simulink model "CRCL"  (R2020b)
settings: Solver=FixedStepDiscrete  StartTime=0.0  StopTime=inf  FixedStep=0.01  RelTol=1e-3  EnableMultiTasking=on
values from neighbouring files (symbols this model uses):
  calibrationDelayTime_s = 2.0    [CRCL_Dictionary.sldd]
  collisionAngleThreshold_deg = 40.0    [CRCL_Dictionary.sldd]
  collisionVarianceThreshold_g2 = 8.0    [CRCL_Dictionary.sldd]
  cpMaxAbortTime_s = 30.0    [CRCL_Dictionary.sldd]
  cpMaxTipOverAngle_deg = 35.0    [CRCL_Dictionary.sldd]
  cpMinEstDistance_m = 50.0    [CRCL_Dictionary.sldd]
  cpMinEstDistanceGnssBased_m = 200.0    [CRCL_Dictionary.sldd]
  cpMinRiddenTime_s = 15.0    [CRCL_Dictionary.sldd]
  cpMinSpeedRiding_kmh = 10.0    [CRCL_Dictionary.sldd]
  cpNumCrankRevolutionThreshold = 5.0    [CRCL_Dictionary.sldd]
  cpSpeedCond2PositiveSpeedChangeTime_s = 5.0    [CRCL_Dictionary.sldd]
  cpSpeedDerivativeThreshold_kmhs = 0.005    [CRCL_Dictionary.sldd]
  cpTimeOutSpeedCond2_s = 15.0    [CRCL_Dictionary.sldd]
  groundHitEnergyThresholdStanding_g2s2 = 0.02    [CRCL_Dictionary.sldd]
  groundHitTipOverAngleThreshold_deg = 40.0    [CRCL_Dictionary.sldd]
  longAccCompForEulerEstFlag = 0.0    [CRCL_Dictionary.sldd]
  minEnergyStrongHit_g2s2 = 0.1    [CRCL_Dictionary.sldd]
  noMotionAccVarianceThresholdSD_g2 = 0.001    [CRCL_Dictionary.sldd]
  ride1minSpeedSlow_kmh = 4.0    [CRCL_Dictionary.sldd]
  ride2minSpeed_kmh = 8.0    [CRCL_Dictionary.sldd]
  rroMaxSpeed_kmh = 5.0    [CRCL_Dictionary.sldd]
  rroMinGyrX_degs = 20.0    [CRCL_Dictionary.sldd]
  rroMonotonyThreshold_degs = -1.0    [CRCL_Dictionary.sldd]
  rroRollIntegrationAngleThreshold_degs = 20.0    [CRCL_Dictionary.sldd]
  rroUniContinuityThreshold_degs = 15.0    [CRCL_Dictionary.sldd]
  scaleFactorVarianceStrongHit = 2.0    [CRCL_Dictionary.sldd]
  sdoMaxAccVarFreeFall_g2 = 0.06    [CRCL_Dictionary.sldd]
  sdoMaxTipOverAngle_deg = 20.0    [CRCL_Dictionary.sldd]
  sdoMinAccVar_g2 = 8.0    [CRCL_Dictionary.sldd]
  sdoMinGyrXYNorm_degs = 720.0    [CRCL_Dictionary.sldd]
  sdoMinGyrXYNormFreeFall_degs = 100.0    [CRCL_Dictionary.sldd]
  sdoMinOrientationChange_deg = 120.0    [CRCL_Dictionary.sldd]
  sdoScaleFactorOrientationChange = 3.0    [CRCL_Dictionary.sldd]
  stepTime_s = 0.01    [CRCL_Dictionary.sldd]
  strongHitSafetyFactor = 2.5    [CRCL_Dictionary.sldd]
  tipOverAccZFiltTreshold_g = 0.7    [CRCL_Dictionary.sldd]
  tipOverAngleThreshold_deg = 50.0    [CRCL_Dictionary.sldd]
  tipOverMinAccZFiltNoseOver_g = 0.3    [CRCL_Dictionary.sldd]
  tipOverRollPitchRelationNoseOver = 1.5    [CRCL_Dictionary.sldd]
undefined symbols (not defined in the file or in its folder): magnitude
libraries: simulink x17
(part 7 of 8)

== matlab function CRCL/MATLAB Function5 ==
  data: tipOverAngle_deg input; probCollision output; probStrongCollision output; probSoftCollision output; speed_kmh input; accEnergyXY50ms input; accEnergyXY70ms input; accEnergyXY70msLatched input; accVariance70msLatched input; secondCalibDone input; probGroundHit output; accImpulseY input; RollDeriv input; probRd1 output; probRd2 output; probTipOver12 output; probTipOver2 output; speedDerivative input; tipOverAngleTransformedColl output; speedTransformedColl output; speed2sTransformedRd output; speedDerivativeTransformedRd output; accTipOverAngle_deg input; pitch_deg input; roll_deg input; accBfZfilt input; tipOverAngleFusedTransformedTOl output; TipOverAngleAccTransformedTOl output; pitchAngleTransformationTO2 output; pitchRollRelationTransformationTO2 output; accBfZTransformationTO2 output; systemConfig input; cobiHubSetup input; curDuAccZFiltG input
function [probCollision, probStrongCollision, probSoftCollision, ...
    probGroundHit, probRd1, probRd2, probTipOver12, probTipOver2, ...
    tipOverAngleTransformedColl, speedTransformedColl,...
    speed2sTransformedRd, speedDerivativeTransformedRd,...
    tipOverAngleFusedTransformedTOl, TipOverAngleAccTransformedTOl , ...
    pitchAngleTransformationTO2, pitchRollRelationTransformationTO2, ...
    accBfZTransformationTO2] = crashFeatureProbabilityEstimation(tipOverAngle_deg, ...
    speed_kmh, accEnergyXY50ms, accEnergyXY70ms, accEnergyXY70msLatched,...
    accVariance70msLatched, secondCalibDone, ...
    accImpulseY,RollDeriv, speedDerivative, accTipOverAngle_deg, ...
    pitch_deg, roll_deg, accBfZfilt, systemConfig, cobiHubSetup, ...
    curDuAccZFiltG)

persistent i ringBufSpeed2s speed2s_kmh

if isempty(i)
    i = single(1);
    ringBufSpeed2s= single(zeros(20,1));
    speed2s_kmh = single(0);  
end

if mod(i,10) == 0
    ringBufSpeed2s(i/10) = speed_kmh;
    if i == 200
        speed2s_kmh = ringBufSpeed2s(1);
    else
        speed2s_kmh = ringBufSpeed2s(i/10+1);
    end
    if min(ringBufSpeed2s) < speed2s_kmh
        speed2s_kmh = min(ringBufSpeed2s);
    end
end


%% general parameters
strongCollisionSafety = single(3);
softCollisionScale = single(2);


%% probabilistic models
B_groundHit = single([-32.0602312846622;30.8165649192532;0.531118388570848;172.376443479951]);
B_collision = single([-2.87196689910160;-29.6105557448201;-5.00762861256094;241.946430188289]);
B_rd1 = single([-29.0217184513153;8.06889061930136]);
B_rd2 = single([-42.1335668740954;23.9784829246872;9.23975798539886;1.14044463386772]);
%B_tipOver12 = single([-1.371493988037109e+02;68.892066955566400;74.731811523437500]);
B_tipOver12 = single([-32.032394409179690;21.612045288085938;19.315736770629883]);
B_tipOver2 =single([-31.113632202148438;15.738595962524414;10.099098205566406;12.869010925292969]);


%% variable transformation
% CollisionHit and GroundHit
% speed:   'f(x)=1-exp(-speedTransform_c0*x)'
c0_speedTransformColl = 0.125;

speedTransformedColl = 1-expApproxFunc(-c0_speedTransformColl*speed_kmh);

% tipOverAngleSigmoid:
% 'f(x)=1/(1+expApproxFunc(-tipOverTransform_c0*(x-tipOverTransform_c1)))'
tipOverSigmoidTransformColl_c0 = single(0.3);   %0.4
tipOverSigmoidTransformColl_c1 = single(42);    %38

tipOverAngleTransformedColl = 1/(1+expApproxFunc(-tipOverSigmoidTransformColl_c0*(tipOverAngle_deg-tipOverSigmoidTransformColl_c1)));

% TipOverFeature
tipOverSigmoidTransformTol_c0 = single(0.33); %0.5
tipOverSigmoidTransformTol_c1 = single(45); 
noseOverSigmoidTransformTo2_c0 = single(0.1); %0.5
noseOverSigmoidTransformTo2_c1 = single(45); 
noseOverSigmoidAccTransform_c0 = 50;
noseOverSigmoidAccTransform_c1 = 0.3;
noseOverSigmoidPitchRollRelationTransform_c0 = 10;
noseOverSigmoidPitchRollRelationTransform_c1 = 1.5;


tipOverAngleFusedTransformedTOl = 1/(1+expApproxFunc(-tipOverSigmoidTransformTol_c0*(tipOverAngle_deg-tipOverSigmoidTransformTol_c1)));
TipOverAngleAccTransformedTOl = 1/(1+expApproxFunc(-tipOverSigmoidTransformTol_c0*(accTipOverAngle_deg-tipOverSigmoidTransformTol_c1)));
pitchAngleTransformationTO2= 1/(1+expApproxFunc(-noseOverSigmoidTransformTo2_c0*(pitch_deg-noseOverSigmoidTransformTo2_c1)));
pitchRollRelationTransformationTO2 = 1/(1+expApproxFunc(-noseOverSigmoidPitchRollRelationTransform_c0*(abs(pitch_deg)/abs(roll_deg)-noseOverSigmoidPitchRollRelationTransform_c1)));
accBfZTransformationTO2 = 1/(1+expApproxFunc(-noseOverSigmoidAccTransform_c0*(accBfZfilt-noseOverSigmoidAccTransform_c1)));

% RideFeature
%speed(t-2s)
c0_SpeedTransformRd = single(5); 
c1_SpeedTransformRd = single(8);

speed2sTransformedRd = 1./(1+expApproxFunc(-c0_SpeedTransformRd.*(speed2s_kmh-c1_SpeedTransformRd)));

%speed derivative
c0_SpeedDerivativeTransformRd = single(10); 
c1_SpeedDerivativeTransformRd = single(-2.5); 

speedDerivativeTransformedRd = 1./(1+expApproxFunc(-c0_SpeedDerivativeTransformRd.*(speedDerivative-c1_SpeedDerivativeTransformRd)));

%% estimation of crash feature probabilities

if secondCalibDone == 1
    %collision
    if accEnergyXY70ms >= 0.003 && tipOverAngle_deg <= 45
        probCollision = 1 ./ (1 + expApproxFunc(-(B_collision(1) + ...
            tipOverAngleTransformedColl .* B_collision(2) + speedTransformedColl .* ...
            B_collision(3) + accEnergyXY70ms .* B_collision(4)))); %sigmoid function
    else
        probCollision = single(0);
    end

    %strongCollision
    if accEnergyXY70msLatched >= 0.003 && tipOverAngle_deg <= 45 && ...
            accVariance70msLatched >= 12                                    %min variance for strongHits!
        probStrongCollision = 1 ./ (1 + expApproxFunc(-(B_collision(1) + ...
            tipOverAngleTransformedColl .* B_collision(2) + speedTransformedColl .* ...
            B_collision(3) + 1/strongCollisionSafety * accEnergyXY70msLatched .* B_collision(4)))); %sigmoid function
    else
        probStrongCollision = single(0);
    end

    %softCollision
    if accEnergyXY70ms >= 0.003 && tipOverAngle_deg <= 45 && speed_kmh <= 4.5 && ...
            (accImpulseY*RollDeriv >= 0 || accEnergyXY70ms >= 0.015 || tipOverAngle_deg <= 10)  % dismiss fallOver on pedal
        probSoftCollision = 1 ./ (1 + expApproxFunc(-(B_collision(1) + ...
            tipOverAngleTransformedColl .* B_collision(2) + speedTransformedColl .* ...
            B_collision(3) + softCollisionScale * accEnergyXY70ms .* B_collision(4)))); %sigmoid function
    else
        probSoftCollision = single(0);
    end

    %groundHit
    if accEnergyXY50ms >= 0.002 && tipOverAngle_deg >= 35
        probGroundHit = 1 ./ (1 + expApproxFunc(-(B_groundHit(1) + ...
            tipOverAngleTransformedColl .* B_groundHit(2) + speedTransformedColl .* ...
            B_groundHit(3) + accEnergyXY50ms .* B_groundHit(4)))); %sigmoid function
    else
        probGroundHit = single(0);
    end
    
    %tipOver Feature
    if systemConfig == 2 && cobiHubSetup == 2 && curDuAccZFiltG <= 0.75
        probTipOver12 = single(1 ./ (1 + expApproxFunc(-(B_tipOver12(1) + ...
            tipOverAngleFusedTransformedTOl .* B_tipOver12(2) + ...
            TipOverAngleAccTransformedTOl .* B_tipOver12(3)))));
    elseif systemConfig ~= 2 || cobiHubSetup ~= 2
        probTipOver12 = single(1 ./ (1 + expApproxFunc(-(B_tipOver12(1) + ...
            tipOverAngleFusedTransformedTOl .* B_tipOver12(2) + ...
            TipOverAngleAccTransformedTOl .* B_tipOver12(3)))));
    else
        probTipOver12 = single(0);
    end
    if abs(roll_deg) <= 30
        probTipOver2 = single(1 ./ (1 + expApproxFunc(-(B_tipOver2(1) + ...
            pitchAngleTransformationTO2 .* B_tipOver2(2) + ...
            pitchRollRelationTransformationTO2 .* B_tipOver2(3)+ ...
             accBfZTransformationTO2 .* B_tipOver2(4)))));
    else
        probTipOver2 = single(0);
    end
    
else    
    %no Calibration yet
    probCollision = single(0);
    probStrongCollision = single(0);
    probSoftCollision = single(0);
    probGroundHit = single(0);
    probTipOver12 = single(0);
    probTipOver2 = single(0);
end

%Ride Feature
probRd1 = 1./(1+expApproxFunc(-(B_rd1(1)+B_rd1(2).*speed_kmh)));
probRd2 = 1 ./ (1 + expApproxFunc(-(B_rd2(1) + speed2sTransformedRd .* B_rd2(2) + ...
    speedDerivativeTransformedRd .* B_rd2(3) + speed_kmh .* B_rd2(4)))); %sigmoid function


speed2sDebug_kmh = speed2s_kmh;

i = i + 1;
if i >= 201
    i=single(1);
end

end

%approximation for exponential function
function y = expApproxFunc(x_arg)

    denominatorPower = single(1024);
    log2Denominator = single(10);

    expApprox = 1+x_arg/denominatorPower;

    for i=1:log2Denominator
        expApprox = expApprox.*expApprox;
    end
    
    y = expApprox;
end

== stateflow chart CRCL/Chart3 ==
  state accXYEnergy70ms [parallel]
    settings: executionOrder=1
    state Latch
      entry:
    state Idle
      entry:
      LF_accXYEnergy70msLatched = LF_curAccXYEnergy70ms;
      during:
      LF_accXYEnergy70msLatched = LF_curAccXYEnergy70ms;
    (default) -> accXYEnergy70ms.Idle
    accXYEnergy70ms.Idle -> accXYEnergy70ms.Latch : [LF_curAccXYEnergy70ms >= 0.01]
        | {
        | LF_accXYEnergy70msLatched = LF_curAccXYEnergy70ms;
        | }
    accXYEnergy70ms.Latch -> accXYEnergy70ms.Latch [order 2] : [LF_accXYEnergy70msLatched < LF_curAccXYEnergy70ms]
        | {
        | LF_accXYEnergy70msLatched = LF_curAccXYEnergy70ms;
        | }
    accXYEnergy70ms.Latch -> accXYEnergy70ms.Idle [order 1] : [after(0.2,sec)]
    accXYEnergy70ms.Latch -> accXYEnergy70ms.Latch [order 3] : [LF_curAccXYEnergy70ms > 0.02]
  state accXYVariance70ms [parallel]
    settings: executionOrder=2
    state Latch
      entry:
    state Idle
      entry:
      LF_accVariance70msLatched = LF_curAccVariance70ms;
      during:
      LF_accVariance70msLatched = LF_curAccVariance70ms;
    (default) -> accXYVariance70ms.Idle
    accXYVariance70ms.Idle -> accXYVariance70ms.Latch : [LF_curAccVariance70ms >= 5]
        | {
        | LF_accVariance70msLatched = LF_curAccVariance70ms;
        | }
    accXYVariance70ms.Latch -> accXYVariance70ms.Latch [order 2] : [LF_accVariance70msLatched < LF_curAccVariance70ms]
        | {
        | LF_accVariance70msLatched = LF_curAccVariance70ms;
        | }
    accXYVariance70ms.Latch -> accXYVariance70ms.Idle [order 1] : [after(0.2,sec)]
    accXYVariance70ms.Latch -> accXYVariance70ms.Latch [order 3] : [LF_curAccVariance70ms > 5]
  state tipOverAngleFused [parallel]
    settings: executionOrder=3
    state Latch
      entry:
    state Idle
      entry:
      LF_tipOverAngleFusedLatched = LF_tipOverAngleFused;
      during:
      LF_tipOverAngleFusedLatched = LF_tipOverAngleFused;
    (default) -> tipOverAngleFused.Idle
    tipOverAngleFused.Idle -> tipOverAngleFused.Latch : [LF_tipOverAngleFused >= 45]
        | {
        | LF_tipOverAngleFusedLatched = LF_tipOverAngleFused;
        | }
    tipOverAngleFused.Latch -> tipOverAngleFused.Latch [order 2] : [LF_tipOverAngleFusedLatched < LF_tipOverAngleFused]
        | {
        | LF_tipOverAngleFusedLatched = LF_tipOverAngleFused;
        | }
    tipOverAngleFused.Latch -> tipOverAngleFused.Idle [order 1] : [after(3,sec)]
    tipOverAngleFused.Latch -> tipOverAngleFused.Latch [order 3] : [LF_tipOverAngleFused > 45]
  data: LF_curAccVariance70ms input; LF_curAccXYEnergy70ms input; LF_accXYEnergy70msLatched output; LF_accVariance70msLatched output; LF_tipOverAngleFused input; LF_tipOverAngleFusedLatched output

== matlab function CRCL/FilterButterworth/MATLAB Function ==
  data: input input; output output
function output = variabelRateLimiter(input)

persistent lastOutput

if isempty(lastOutput)
   lastOutput = single(0); 
end

if input >= lastOutput || lastOutput <= 0.4 || 1/15*(lastOutput-input) <= 0.025
    output = input;
else
    if 1/5*(lastOutput-input) > 0.4
        output = lastOutput-1/5*(lastOutput-input);
    else
        output = lastOutput-1/15*(lastOutput-input);
    end
end

lastOutput = output;
end

== stateflow chart CRCL/Chart1 ==
  state EstimateLongitudinalAcceleration [parallel]
    settings: executionOrder=1
    state speedChange
      en:
      if LAE_timer_s < 2 && LAE_timer_s > 0 % AVOID DIVISION BY ZERO!
      LAE_longAccTmp_g = (LAE_curSpeed_kmh-LAE_lastSpeed_kmh)/(3.6*9.81*LAE_timer_s);
      else
      LAE_longAccTmp_g = (LAE_curSpeed_kmh-LAE_lastSpeed_kmh)/(3.6*9.81);
      end
      LAE_lastSpeed_kmh = LAE_curSpeed_kmh;
      LAE_timerReset = int16(1);
      if LAE_longAccTmp_g > LAE_curAccBfXFilt_g && LAE_curAccBfXFilt_g > 0 && LAE_longAccTmp_g > 0
      LAE_longAcc_g = LAE_curAccBfXFilt_g;
      elseif LAE_longAccTmp_g < LAE_curAccBfXFilt_g && LAE_curAccBfXFilt_g < 0 && LAE_longAccTmp_g < 0
      LAE_longAcc_g = LAE_curAccBfXFilt_g;
      elseif int8(sign(LAE_curAccBfXFilt_g)) ~= int8(sign(LAE_longAccTmp_g))
      LAE_longAcc_g = single(0);
      else
      LAE_longAcc_g = LAE_longAccTmp_g;
      end
      du:
      %if filtered accX signal is still changing
      if LAE_longAccTmp_g > LAE_curAccBfXFilt_g && LAE_curAccBfXFilt_g > 0 && LAE_longAccTmp_g > 0
      LAE_longAcc_g = LAE_curAccBfXFilt_g;
      elseif LAE_longAccTmp_g < LAE_curAccBfXFilt_g && LAE_curAccBfXFilt_g < 0 && LAE_longAccTmp_g < 0
      LAE_longAcc_g = LAE_curAccBfXFilt_g;
      elseif int8(sign(LAE_curAccBfXFilt_g)) ~= int8(sign(LAE_longAccTmp_g))
      LAE_longAcc_g = single(0);
      else
      LAE_longAcc_g = LAE_longAccTmp_g;
      end
    state Idle
      du:
      LAE_lastSpeed_kmh = LAE_curSpeed_kmh;
    (default) -> Idle : {
        | LAE_lastSpeed_kmh = single(0);
        | LAE_longAcc_g = single(0);
        | LAE_longAccTmp_g = single(0);
        | }
    speedChange -> speedChange [commented out] : %accelerating
        | [LAE_curSpeed_kmh-LAE_lastSpeed_kmh > LAE_minSpeedDelta_kmh && ...
        |  LAE_lastSpeed_kmh >= LAE_minSpeed_kmh && ...
        | LAE_curCalibState == 1]
    speedChange -> speedChange [commented out] : %decelerating
        | [LAE_lastSpeed_kmh-LAE_curSpeed_kmh > LAE_minSpeedDelta_kmh && ...
        | (LAE_curSpeed_kmh >= LAE_minSpeed_kmh || ...
        |  LAE_lastSpeed_kmh >= LAE_minSpeed_kmh) && ...
        | LAE_curCalibState == 1]
    Idle -> speedChange [commented out] : %decelerating
        | [LAE_lastSpeed_kmh-LAE_curSpeed_kmh > LAE_minSpeedDelta_kmh && ...
        | (LAE_curSpeed_kmh >= LAE_minSpeed_kmh || ...
        |  LAE_lastSpeed_kmh >= LAE_minSpeed_kmh) && ...
        | LAE_curCalibState == 1]
    Idle -> speedChange [commented out] : %accelerating
        | [LAE_curSpeed_kmh-LAE_lastSpeed_kmh > LAE_minSpeedDelta_kmh && ...
        |  LAE_lastSpeed_kmh >= LAE_minSpeed_kmh && ...
        | LAE_curCalibState == 1]
    Idle -> speedChange : [abs(LAE_curSpeed_kmh-LAE_lastSpeed_kmh) > LAE_minSpeedDelta_kmh && ...
        |  (LAE_curSpeed_kmh >= LAE_minSpeed_kmh || ...
        |  LAE_lastSpeed_kmh >= LAE_minSpeed_kmh) && ...
        | LAE_curCalibState == 1]
    speedChange -> Idle [order 2] : [after(1.05,sec)] %GPS speed rate ~1Hz
        | {
        | LAE_longAcc_g = single(0);
        | LAE_longAccTmp_g = single(0);
        | }
    speedChange -> speedChange [order 1] : [abs(LAE_curSpeed_kmh-LAE_lastSpeed_kmh) > LAE_minSpeedDelta_kmh && ...
        |  (LAE_curSpeed_kmh >= LAE_minSpeed_kmh || ...
        |  LAE_lastSpeed_kmh >= LAE_minSpeed_kmh) && ...
        | LAE_curCalibState == 1]
  state SpeedUpdateTime [parallel]
    settings: executionOrder=2
    state Counter
      en:
      LAE_timer_s = single(0);
      LAE_timerReset = int16(0);
      du:
      LAE_timer_s = LAE_timer_s + LAE_timeStep_s;
    (default) -> Counter
    Counter -> Counter : [LAE_timerReset == 1]
  data: LAE_minSpeed_kmh input; LAE_curSpeed_kmh input; LAE_minSpeedDelta_kmh input; LAE_longAcc_g output; LAE_lastSpeed_kmh local; LAE_curAccBfXFilt_g input; LAE_longAccTmp_g output; LAE_curCalibState input; LAE_timeStep_s input; LAE_timerReset local; LAE_timer_s output

== stateflow chart CRCL/Chart2 ==
  state TimeOutVariables [parallel]
    settings: executionOrder=2
    state Iinitialze
      entry:
      LP_timeOutRide1 = single(5);
      LP_timeOutColl = single(5);
      LP_timeOutTipOver = single(2);
      LP_timeOutGroundHit = single(3.5);
    (default) -> Iinitialze
  state Ride1 [parallel]
    settings: executionOrder=1
    state Latch
      entry:
    state Idle
      entry:
      LP_probRide1Latched = LP_curProbRide1;
      during:
      LP_probRide1Latched = LP_curProbRide1;
    (default) -> Ride1.Idle
    Ride1.Idle -> Ride1.Latch : [LP_curProbRide1 >= 0.9]
        | {
        | LP_probRide1Latched = LP_curProbRide1;
        | }
    Ride1.Latch -> Ride1.Latch [order 2] : [LP_probRide1Latched < LP_curProbRide1]
        | {
        | LP_probRide1Latched = LP_curProbRide1;
        | }
    Ride1.Latch -> Ride1.Idle [order 1] : [after(LP_timeOutRide1,sec)]
    Ride1.Latch -> Ride1.Latch [order 3] : [LP_curProbRide1 > 0.9]
  state TipOver [parallel]
    settings: executionOrder=7
    state Latch
      entry:
      LP_probTipOverTimer = LP_probTipOverTimer + 1;
      du:
      LP_probTipOverTimer = LP_probTipOverTimer + 1;
    state Idle
      entry:
      LP_probTipOverLatched = LP_curProbTipOver;
      LP_probTipOverTimer = uint16(0);
      during:
      LP_probTipOverLatched = LP_curProbTipOver;
    (default) -> TipOver.Idle
    TipOver.Idle -> TipOver.Latch : [LP_curProbTipOver >= 0.2]
        | {
        | LP_probTipOverLatched = LP_curProbTipOver;
        | }
    TipOver.Latch -> TipOver.Latch [order 1] : [LP_probTipOverLatched < LP_curProbTipOver]
        | {
        | LP_probTipOverLatched = LP_curProbTipOver;
        | }
    TipOver.Latch -> TipOver.Idle [order 2] : [after(LP_timeOutTipOver,sec)]
    TipOver.Latch -> TipOver.Latch [order 3] : [LP_curProbTipOver > 0.9]
  state Ride2 [parallel]
    settings: executionOrder=3
    state Idle
      entry:
      LP_probRide2Latched = LP_curProbRide2;
      during:
      LP_probRide2Latched = LP_curProbRide2;
    (default) -> Ride2.Idle
  state NoseOver [parallel]
    settings: executionOrder=8
    state Latch
      entry:
    state Idle
      entry:
      LP_probNoseOverLatched = LP_curProbNoseOver;
      during:
      LP_probNoseOverLatched = LP_curProbNoseOver;
    (default) -> NoseOver.Idle
    NoseOver.Idle -> NoseOver.Latch : [LP_curProbNoseOver >= 0.2]
        | {
        | LP_probNoseOverLatched = LP_curProbNoseOver;
        | }
    NoseOver.Latch -> NoseOver.Latch [order 1] : [LP_probNoseOverLatched < LP_curProbNoseOver]
        | {
        | LP_probNoseOverLatched = LP_curProbNoseOver;
        | }
    NoseOver.Latch -> NoseOver.Idle [order 3] : [after(LP_timeOutTipOver,sec)]
    NoseOver.Latch -> NoseOver.Latch [order 2] : [LP_curProbTipOver > 0.9]
  state Collision [parallel]
    settings: executionOrder=4
    state Latch
      entry:
    state Idle
      entry:
      LP_probCollLatched = LP_curProbColl;
      during:
      LP_probCollLatched = LP_curProbColl;
    (default) -> Collision.Idle
    Collision.Idle -> Collision.Latch : [LP_curProbColl >= 0.2 && LP_bikeUpright == 1]
        | {
        | LP_probCollLatched = LP_curProbColl;
        | }
    Collision.Latch -> Collision.Latch [order 2] : [LP_probCollLatched < LP_curProbColl && LP_bikeUpright == 1]
        | {
        | LP_probCollLatched = LP_curProbColl;
        | }
    Collision.Latch -> Collision.Idle [order 1] : [after(LP_timeOutColl,sec)]
  state GroundHit [parallel]
    settings: executionOrder=9
    state Idle
      entry:
      LP_probGroundHitLatched = LP_curProbGroundHit;
      during:
      LP_probGroundHitLatched = LP_curProbGroundHit;
    state Latch
      entry:
    (default) -> GroundHit.Idle
    GroundHit.Idle -> GroundHit.Latch : [LP_curProbGroundHit >= 0.2]
        | {
        | LP_probGroundHitLatched = LP_curProbGroundHit;
        | }
    GroundHit.Latch -> GroundHit.Latch [order 2] : [LP_probGroundHitLatched < LP_curProbGroundHit]
        | {
        | LP_probGroundHitLatched = LP_curProbGroundHit;
        | }
    GroundHit.Latch -> GroundHit.Idle [order 1] : [after(LP_timeOutGroundHit,sec)]
  state SoftCollision [parallel]
    settings: executionOrder=5
    state Latch
      entry:
    state Idle
      entry:
      LP_probSoftCollLatched = LP_curProbSoftColl;
      during:
      LP_probSoftCollLatched = LP_curProbSoftColl;
    (default) -> SoftCollision.Idle
    SoftCollision.Idle -> SoftCollision.Latch : [LP_curProbSoftColl >= 0.2 && LP_bikeUpright == 1]
        | {
        | LP_probSoftCollLatched = LP_curProbSoftColl;
        | }
    SoftCollision.Latch -> SoftCollision.Latch [order 2] : [LP_probSoftCollLatched < LP_curProbSoftColl && LP_bikeUpright == 1]
        | {
        | LP_probSoftCollLatched = LP_curProbSoftColl;
        | }
    SoftCollision.Latch -> SoftCollision.Idle [order 1] : [after(LP_timeOutColl,sec)]
  state Ride3 [parallel]
    settings: executionOrder=10
    state latching
      entry:
      LP_probRroLatched = LP_curProbRro;
    state Idle
      entry:
      LP_probRroLatched = LP_curProbRro;
      during:
      LP_probRroLatched = LP_curProbRro;
    (default) -> Ride3.Idle
    Ride3.Idle -> latching : [LP_curProbRro > 0.5 && LP_curProbTipOver > 0.5]
    latching -> Ride3.Idle : [LP_curProbRro < 0.5 && LP_probTipOverLatched < 0.5]
  state StrongCollision [parallel]
    settings: executionOrder=6
    state Latch
      entry:
    state Idle
      entry:
      LP_probStrongCollLatched = LP_curProbStrongColl;
      during:
      LP_probStrongCollLatched = LP_curProbStrongColl;
    (default) -> StrongCollision.Idle
    StrongCollision.Idle -> StrongCollision.Latch : [LP_curProbStrongColl >= 0.2 && LP_bikeUpright == 1]
        | {
        | LP_probStrongCollLatched = LP_curProbStrongColl;
        | }
    StrongCollision.Latch -> StrongCollision.Latch [order 2] : [LP_probStrongCollLatched < LP_curProbStrongColl && LP_bikeUpright == 1]
        | {
        | LP_probStrongCollLatched = LP_curProbStrongColl;
        | }
    StrongCollision.Latch -> StrongCollision.Idle [order 1] : [after(LP_timeOutColl,sec)]
  data: LP_curProbColl input; LP_curProbSoftColl input; LP_curProbGroundHit input; LP_curProbStrongColl input; LP_curProbRide1 input; LP_curProbNoseOver input; LP_curProbRide2 input; LP_curProbTipOver input; LP_probRide2Latched output; LP_probGroundHitLatched output; LP_probSoftCollLatched output; LP_probCollLatched output; LP_probStrongCollLatched output; LP_timeOutTipOver local; LP_probRide1Latched output; LP_timeOutRide1 local; LP_timeOutColl local; LP_timeOutGroundHit local; LP_probTipOverLatched output; LP_probNoseOverLatched output; LP_curProbRro input; LP_probRroLatched output; LP_probTipOverTimer output; LP_bikeUpright input
